simulink model "proj2"  (R2018b)
settings: Solver=ode4  StartTime=0.0  StopTime=0.12  FixedStep=0.0001  RelTol=1e-3
values from neighbouring files (symbols this model uses):
  alpha = atan(wL_es/r_s)    [arb_ref_frame.m]
  scale = system{kk}{2}    [arb_ref_frame.m]
  tau = L_s/r_s    (= 0.0133854013164)    [arb_ref_frame.m]
  test_case = jj    [arb_ref_frame.m]
  v_s = 10/sqrt(2)    [arb_ref_frame.m]
  w_e = 377    [arb_ref_frame.m]
  z_s = r_s + 1j*wL_es    [arb_ref_frame.m]
libraries: simulink x1
settings Model: Creator=carlo  LastModifiedBy=carlo

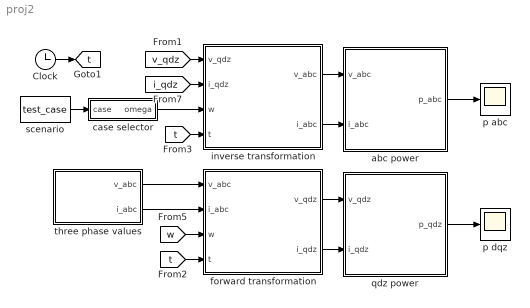
== system proj2 ==
  Clock : Clock
  abc power : Subsystem
  case selector : Subsystem
  forward transformation : Subsystem
  inverse transformation : Subsystem
  p abc : Scope
  p dqz : Scope
  qdz power : Subsystem
  scenario : Constant  Value=test_case
  three phase values : Subsystem
  tag scope: t=global
  wires:
  scenario/1 -> case selector/1(case)
  three phase values/1(v_abc) -> forward transformation/1(v_abc)
  three phase values/2(i_abc) -> forward transformation/2(i_abc)
  [w] -> forward transformation/3(w)
  [t] -> forward transformation/4(t)
  [v_qdz] -> inverse transformation/1(v_qdz)
  [i_qdz] -> inverse transformation/2(i_qdz)
  case selector/1(omega) -> inverse transformation/3(w)
  [t] -> inverse transformation/4(t)
  inverse transformation/1(v_abc) -> abc power/1(v_abc)
  inverse transformation/2(i_abc) -> abc power/2(i_abc)
  abc power/1(p_abc) -> p abc/1
  forward transformation/1(v_qdz) -> qdz power/1(v_qdz)
  forward transformation/2(i_qdz) -> qdz power/2(i_qdz)
  qdz power/1(p_qdz) -> p dqz/1
  Clock/1 -> [t]

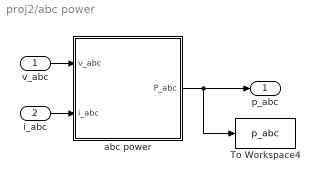
== system proj2/abc power ==
  v_abc : Inport
  i_abc : Inport  Port=2
  To Workspace4 : ToWorkspace  VariableName=p_abc  SaveFormat=Timeseries  SampleTime=-1
  abc power : MATLAB Function  TreatAsAtomicUnit=on
  p_abc : Outport
  wires:
  i_abc/1 -> abc power/2(i_abc)
  abc power/1(P_abc) -> p_abc/1, To Workspace4/1
  v_abc/1 -> abc power/1(v_abc)

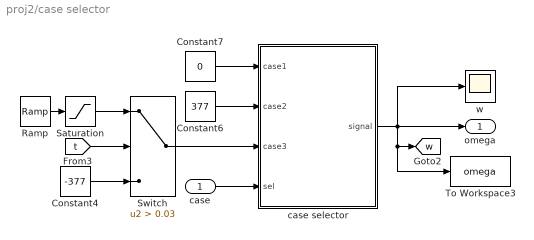
== system proj2/case selector ==
  case : Inport
  Constant4 : Constant  Value=-377
  Constant6 : Constant  Value=377
  Constant7 : Constant  Value=0
  Ramp : simulink/Sources/Ramp  slope=9300  start=ramp_start  InitialOutput=0
  Saturation : Saturate  UpperLimit=377
  Switch : Switch  Criteria=u2 > Threshold  Threshold=0.03
  To Workspace3 : ToWorkspace  VariableName=omega  SaveFormat=Timeseries  SampleTime=-1
  case selector : MATLAB Function  TreatAsAtomicUnit=on
  w : Scope
  omega : Outport
  tag scope: w=global
  wires:
  Saturation/1 -> Switch/1
  Switch/1 -> case selector/3(case3)
  [t] -> Switch/2
  Constant7/1 -> case selector/1(case1)
  Constant6/1 -> case selector/2(case2)
  Ramp/1 -> Saturation/1
  Constant4/1 -> Switch/3
  case/1 -> case selector/4(sel)
  case selector/1(signal) -> w/1, omega/1, [w], To Workspace3/1

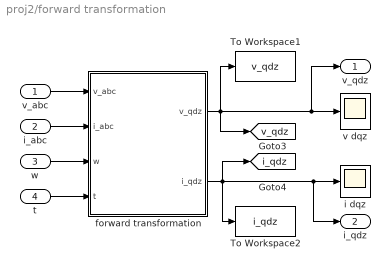
== system proj2/forward transformation ==
  v_abc : Inport
  i_abc : Inport  Port=2
  w : Inport  Port=3
  t : Inport  Port=4
  To Workspace1 : ToWorkspace  VariableName=v_qdz  SaveFormat=Timeseries  SampleTime=-1
  To Workspace2 : ToWorkspace  VariableName=i_qdz  SaveFormat=Timeseries  SampleTime=-1
  forward transformation : MATLAB Function  TreatAsAtomicUnit=on
  i dqz : Scope
  v dqz : Scope
  v_qdz : Outport
  i_qdz : Outport  Port=2
  tag scope: i_qdz=global, v_qdz=global
  wires:
  forward transformation/1(v_qdz) -> [v_qdz], v_qdz/1, v dqz/1, To Workspace1/1
  w/1 -> forward transformation/3(w)
  i_abc/1 -> forward transformation/2(i_abc)
  v_abc/1 -> forward transformation/1(v_abc)
  t/1 -> forward transformation/4(t)
  forward transformation/2(i_qdz) -> [i_qdz], i_qdz/1, i dqz/1, To Workspace2/1

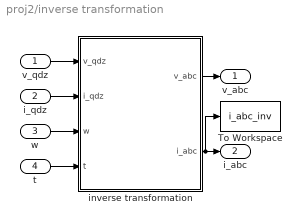
== system proj2/inverse transformation ==
  v_qdz : Inport
  i_qdz : Inport  Port=2
  w : Inport  Port=3
  t : Inport  Port=4
  To Workspace : ToWorkspace  VariableName=i_abc_inv  SaveFormat=Timeseries  SampleTime=-1
  inverse transformation : MATLAB Function  TreatAsAtomicUnit=on
  v_abc : Outport
  i_abc : Outport  Port=2
  wires:
  inverse transformation/2(i_abc) -> To Workspace/1, i_abc/1
  w/1 -> inverse transformation/3(w)
  i_qdz/1 -> inverse transformation/2(i_qdz)
  v_qdz/1 -> inverse transformation/1(v_qdz)
  t/1 -> inverse transformation/4(t)
  inverse transformation/1(v_abc) -> v_abc/1

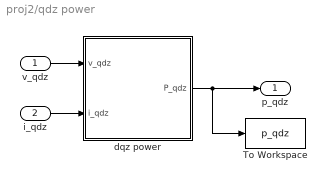
== system proj2/qdz power ==
  v_qdz : Inport
  i_qdz : Inport  Port=2
  To Workspace : ToWorkspace  VariableName=p_qdz  SaveFormat=Timeseries  SampleTime=-1
  dqz power : MATLAB Function  TreatAsAtomicUnit=on
  p_qdz : Outport
  wires:
  dqz power/1(P_qdz) -> p_qdz/1, To Workspace/1
  v_qdz/1 -> dqz power/1(v_qdz)
  i_qdz/1 -> dqz power/2(i_qdz)

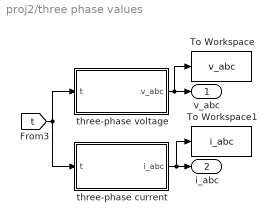
== system proj2/three phase values ==
  To Workspace : ToWorkspace  VariableName=v_abc  SaveFormat=Timeseries  SampleTime=-1
  To Workspace1 : ToWorkspace  VariableName=i_abc  SaveFormat=Timeseries  SampleTime=-1
  three-phase current : MATLAB Function  TreatAsAtomicUnit=on
  three-phase voltage : MATLAB Function  TreatAsAtomicUnit=on
  v_abc : Outport
  i_abc : Outport  Port=2
  wires:
  three-phase voltage/1(v_abc) -> To Workspace/1, v_abc/1
  [t] -> three-phase voltage/1(t), three-phase current/1(t)
  three-phase current/1(i_abc) -> To Workspace1/1, i_abc/1

== matlab function proj2/three phase values/three-phase voltage ==
  data: v_abc output; t input; scale parameter; w_e parameter; v_s parameter
function v_abc = threePhaseV(t, scale, w_e, v_s)
phase = 2*pi/3;
theta = mod(w_e*t, 2*pi);

v_abc = sqrt(2)*v_s*[
    cos(theta);
    scale*cos(theta-phase);
    cos(theta+phase)];

== matlab function proj2/forward transformation/forward transformation ==
  data: v_abc input; i_abc input; w input; t input; v_qdz output; i_qdz output
function [v_qdz,i_qdz]= Ks_forward(v_abc,i_abc,w,t)
phase = 2*pi/3;
theta = mod(w*t, 2*pi);

K_s = (2/3)*[
    cos(theta) cos(theta-phase) cos(theta+phase);
    sin(theta) sin(theta-phase) sin(theta+phase);
    0.5        0.5              0.5];

v_qdz = K_s*v_abc;
i_qdz = K_s*i_abc;

== matlab function proj2/three phase values/three-phase current ==
  data: i_abc output; t input; tau parameter; alpha parameter; z_s parameter; v_s parameter; w_e parameter
function i_abc = threePhaseI(t,tau,alpha, z_s, v_s, w_e)
cf = sqrt(2)*v_s/abs(z_s);
et = -1*exp(-t/tau);
theta = mod(w_e*t, 2*pi);
phase = 2*pi/3;

i_abc = cf*[
    (et*cos(alpha)+cos(theta-alpha));
    (et*cos(alpha+phase)+cos(theta-alpha-phase));
    (et*cos(alpha-phase)+cos(theta-alpha+phase))];

== matlab function proj2/qdz power/dqz power ==
  data: v_qdz input; P_qdz output; i_qdz input
function P_qdz = power(v_qdz,i_qdz)

P_qdz = (3/2)*sum(v_qdz.*i_qdz);

== matlab function proj2/abc power/abc power ==
  data: v_abc input; P_abc output; i_abc input
function P_abc = power(v_abc,i_abc)

P_abc = sum(v_abc.*i_abc);

== matlab function proj2/inverse transformation/inverse transformation ==
  data: v_qdz input; i_qdz input; w input; t input; v_abc output; i_abc output
function [v_abc,i_abc]= Ks_inverse(v_qdz,i_qdz, w,t)
phase = 2*pi/3;
theta = mod(w*t, 2*pi);

K_s_inv = [
    cos(theta)          sin(theta)          1;
    cos(theta-phase)    sin(theta-phase)    1;
    cos(theta+phase)    sin(theta+phase)    1];

v_abc = K_s_inv*v_qdz;
i_abc = K_s_inv*i_qdz;

== matlab function proj2/case selector/case selector ==
  data: case1 input; signal output; case2 input; case3 input; sel input
function signal = case_sel(case1, case2, case3, sel)
switch sel
case 1
    signal = case1;
case 2
    signal = case2;
case 3
    signal = case3;
otherwise
    signal = case1;
end
